simulink model "mpu6050_working"  (R2017a)
settings: Solver=FixedStepDiscrete  StartTime=0.0  StopTime=inf  RelTol=1e-3
PostLoadFcn:
  | ChipSelect = 1;  % choose I2C comms
  | AddressAlt = 0;  % use default address
  | 
  | if AddressAlt == 1
  | % b1101001 (pin AD0 is logic high).
  | SlvAddr = uint8(bin2dec('1101001'));  % ADDR ALT = 1
  | else
  | % b1101000 (pin AD0 is logic low)
  | SlvAddr = uint8(bin2dec('1101000'));  % ADDR ALT = 0
  | end
  | SlvAddr = uint8(hex2dec('68'));
  | 
  | 
  | % 0x3B 59 ACCEL_XOUT[15:8]
  | % 0x3C 60 ACCEL_XOUT[7:0]
  | % 0x3D 61 ACCEL_YOUT[15:8]
  | % 0x3E 62 ACCEL_YOUT[7:0]
  | % 0x3F 63 ACCEL_ZOUT[15:8]
  | % 0x40 64 ACCEL_ZOUT[7:0]
  | 
  | AccelXRegAddr = uint8(hex2dec('3B'));
  | AccelYRegAddr = uint8(hex2dec('3D'));
  | AccelZRegAddr = uint8(hex2dec('3F'));
  | 
  | % 0x43 67 GYRO_XOUT[15:8]
  | % 0x44 68 GYRO_XOUT[7:0]
  | % 0x45 69 GYRO_YOUT[15:8]
  | % 0x46 70 GYRO_YOUT[7:0]
  | % 0x47 71 GYRO_ZOUT[15:8]
  | % 0x48 72 GYRO_ZOUT[7:0]
  | 
  | GyroXRegAddr = uint8(hex2dec('43'));
  | GyroYRegAddr = uint8(hex2dec('45'));
  | GyroZRegAddr = uint8(hex2dec('47'));
  | 
  | deviceAddr = fi(SlvAddr,0,7,0);
  | 
  | powerRegAddr = uint8(hex2dec('6B'));
  | powerRegData = bin2dec('10000001');
undefined symbols (not defined in the file): fpgaClk, Ku, PWMFreq, Tu
libraries: simulink x1
settings Model: DataTypeOverride=Off  Creator=skuznick  LastModifiedBy=mini
settings DataIOCC: SaveOutput=off  SaveTime=off
settings OptimizationCC: BlockReduction=off  ConditionallyExecuteInputs=off  DefaultParameterBehavior=Inlined
settings DebuggingCC: AlgebraicLoopMsg=error  SingleTaskRateTransMsg=error
settings HardwareCC: ProdBitPerPointer=32  ProdBitPerSizeT=32  ProdBitPerPtrDiffT=32  ProdLargestAtomicFloat=None  ProdIntDivRoundTo=Undefined  ProdEndianess=Unspecified  ProdWordSize=32  ProdHWDeviceType=ASIC/FPGA->ASIC/FPGA  ProdEqTarget=off
settings GRTTargetCC: ExtMode=on

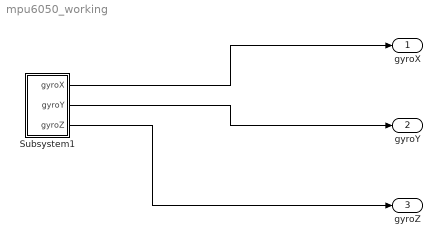
== system mpu6050_working ==
  Subsystem1 : Subsystem
  gyroX : Outport
  gyroY : Outport  Port=2
  gyroZ : Outport  Port=3
  wires:
  Subsystem1/1(gyroX) -> gyroX/1
  Subsystem1/2(gyroY) -> gyroY/1
  Subsystem1/3(gyroZ) -> gyroZ/1

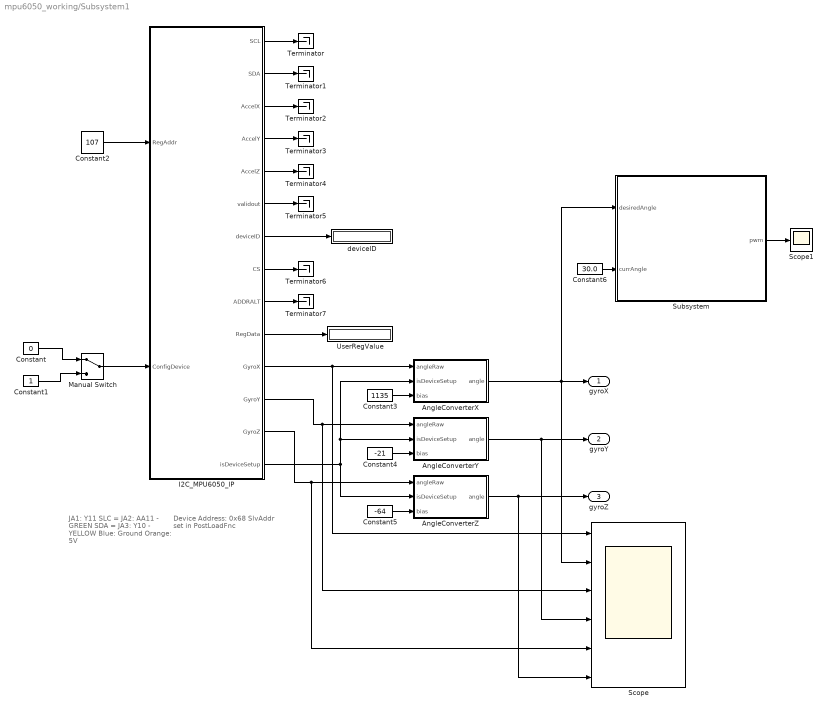
== system mpu6050_working/Subsystem1 ==
  note: JA1: Y11
      | SLC = JA2: AA11 - GREEN
      | SDA = JA3: Y10  - YELLOW
      | Blue: Ground
      | Orange: 5V
  note: Device Address: 0x68
      | SlvAddr set in PostLoadFnc
  AngleConverterX : Subsystem
  AngleConverterY : Subsystem
  AngleConverterZ : Subsystem
  Constant : Constant  Value=0  OutDataTypeStr=boolean  SampleTime=-1
  Constant1 : Constant  OutDataTypeStr=boolean  SampleTime=-1
  Constant2 : Constant  Value=107  OutDataTypeStr=uint8  SampleTime=-1
  Constant3 : Constant  Value=1135  OutDataTypeStr=int16
  Constant4 : Constant  Value=-21  OutDataTypeStr=int16
  Constant5 : Constant  Value=-64  OutDataTypeStr=int16
  Constant6 : Constant  Value=30.0  OutDataTypeStr=double
  I2C_MPU6050_IP : Subsystem  TreatAsAtomicUnit=on  SystemSampleTime=1/400e3
  Manual Switch : ManualSwitch
  Scope : Scope  NumInputPorts=6
  Scope1 : Scope
  Subsystem : Subsystem
  Terminator{,1..7} (8 alike) : Terminator
  UserRegValue : Display
  deviceID : Display
  gyroX : Outport
  gyroY : Outport  Port=2
  gyroZ : Outport  Port=3
  wires:
  I2C_MPU6050_IP/7(deviceID) -> deviceID/1
  Constant/1 -> Manual Switch/1
  Constant1/1 -> Manual Switch/2
  Constant2/1 -> I2C_MPU6050_IP/1(RegAddr)
  I2C_MPU6050_IP/10(RegData) -> UserRegValue/1
  Manual Switch/1 -> I2C_MPU6050_IP/2(ConfigDevice)
  I2C_MPU6050_IP/11(GyroX) -> Scope/1, AngleConverterX/1(angleRaw)
  I2C_MPU6050_IP/12(GyroY) -> Scope/3, AngleConverterY/1(angleRaw)
  Subsystem/1(pwm) -> Scope1/1
  I2C_MPU6050_IP/5(AccelZ) -> Terminator4/1
  AngleConverterZ/1(angle) -> gyroZ/1, Scope/6
  AngleConverterX/1(angle) -> gyroX/1, Subsystem/1(desiredAngle), Scope/2
  I2C_MPU6050_IP/4(AccelY) -> Terminator3/1
  I2C_MPU6050_IP/8(CS) -> Terminator6/1
  I2C_MPU6050_IP/9(ADDRALT) -> Terminator7/1
  Constant6/1 -> Subsystem/2(currAngle)
  I2C_MPU6050_IP/3(AccelX) -> Terminator2/1
  I2C_MPU6050_IP/6(validout) -> Terminator5/1
  I2C_MPU6050_IP/1(SCL) -> Terminator/1
  I2C_MPU6050_IP/2(SDA) -> Terminator1/1
  Constant4/1 -> AngleConverterY/3(bias)
  I2C_MPU6050_IP/14(isDeviceSetup) -> AngleConverterZ/2(isDeviceSetup), AngleConverterY/2(isDeviceSetup), AngleConverterX/2(isDeviceSetup)
  Constant5/1 -> AngleConverterZ/3(bias)
  Constant3/1 -> AngleConverterX/3(bias)
  I2C_MPU6050_IP/13(GyroZ) -> Scope/5, AngleConverterZ/1(angleRaw)
  AngleConverterY/1(angle) -> gyroY/1, Scope/4

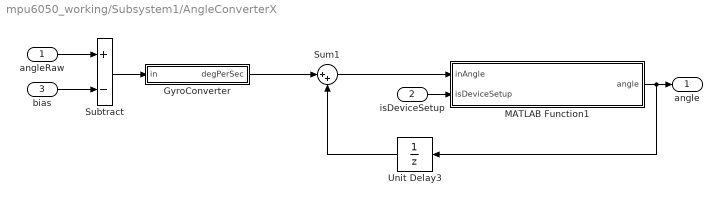
== system mpu6050_working/Subsystem1/AngleConverterX ==
  angleRaw : Inport  OutDataTypeStr=int16  Interpolate=off
  isDeviceSetup : Inport  Port=2  OutDataTypeStr=boolean  Interpolate=off
  bias : Inport  Port=3  OutDataTypeStr=int16  Interpolate=off
  GyroConverter : Subsystem
  MATLAB Function1 : MATLAB Function  TreatAsAtomicUnit=on
  Subtract : Sum  Inputs=+-  OutDataTypeStr=int16  SaturateOnIntegerOverflow=off  InputSameDT=off
  Sum1 : Sum  Inputs=|++  SaturateOnIntegerOverflow=off  InputSameDT=off  OutDataTypeStr=Inherit: Inherit via internal rule
  Unit Delay3 : UnitDelay  SampleTime=-1
  angle : Outport  OutDataTypeStr=double
  wires:
  MATLAB Function1/1(angle) -> Unit Delay3/1, angle/1
  isDeviceSetup/1 -> MATLAB Function1/2(isDeviceSetup)
  Sum1/1 -> MATLAB Function1/1(inAngle)
  Unit Delay3/1 -> Sum1/2
  GyroConverter/1(degPerSec) -> Sum1/1
  angleRaw/1 -> Subtract/1
  bias/1 -> Subtract/2
  Subtract/1 -> GyroConverter/1(in)

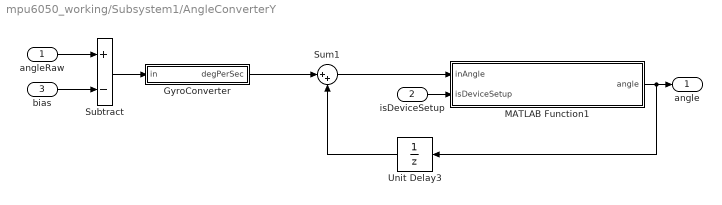
== system mpu6050_working/Subsystem1/AngleConverterY ==
  angleRaw : Inport  OutDataTypeStr=int16  Interpolate=off
  isDeviceSetup : Inport  Port=2  OutDataTypeStr=boolean  Interpolate=off
  bias : Inport  Port=3  OutDataTypeStr=int16  Interpolate=off
  GyroConverter : Subsystem
  MATLAB Function1 : MATLAB Function  TreatAsAtomicUnit=on
  Subtract : Sum  Inputs=+-  OutDataTypeStr=int16  SaturateOnIntegerOverflow=off  InputSameDT=off
  Sum1 : Sum  Inputs=|++  SaturateOnIntegerOverflow=off  InputSameDT=off  OutDataTypeStr=Inherit: Inherit via internal rule
  Unit Delay3 : UnitDelay  SampleTime=-1
  angle : Outport  OutDataTypeStr=double
  wires:
  MATLAB Function1/1(angle) -> Unit Delay3/1, angle/1
  isDeviceSetup/1 -> MATLAB Function1/2(isDeviceSetup)
  Sum1/1 -> MATLAB Function1/1(inAngle)
  Unit Delay3/1 -> Sum1/2
  GyroConverter/1(degPerSec) -> Sum1/1
  angleRaw/1 -> Subtract/1
  bias/1 -> Subtract/2
  Subtract/1 -> GyroConverter/1(in)

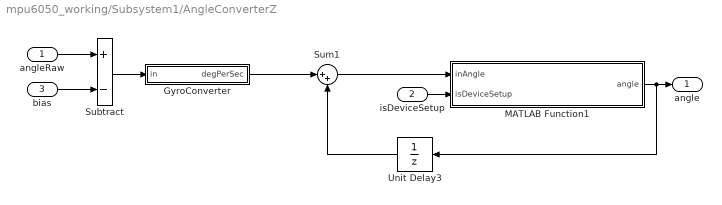
== system mpu6050_working/Subsystem1/AngleConverterZ ==
  angleRaw : Inport  OutDataTypeStr=int16  Interpolate=off
  isDeviceSetup : Inport  Port=2  OutDataTypeStr=boolean  Interpolate=off
  bias : Inport  Port=3  OutDataTypeStr=int16  Interpolate=off
  GyroConverter : Subsystem
  MATLAB Function1 : MATLAB Function  TreatAsAtomicUnit=on
  Subtract : Sum  Inputs=+-  OutDataTypeStr=int16  SaturateOnIntegerOverflow=off  InputSameDT=off
  Sum1 : Sum  Inputs=|++  SaturateOnIntegerOverflow=off  InputSameDT=off  OutDataTypeStr=Inherit: Inherit via internal rule
  Unit Delay3 : UnitDelay  SampleTime=-1
  angle : Outport  OutDataTypeStr=double
  wires:
  MATLAB Function1/1(angle) -> Unit Delay3/1, angle/1
  isDeviceSetup/1 -> MATLAB Function1/2(isDeviceSetup)
  Sum1/1 -> MATLAB Function1/1(inAngle)
  Unit Delay3/1 -> Sum1/2
  GyroConverter/1(degPerSec) -> Sum1/1
  angleRaw/1 -> Subtract/1
  bias/1 -> Subtract/2
  Subtract/1 -> GyroConverter/1(in)

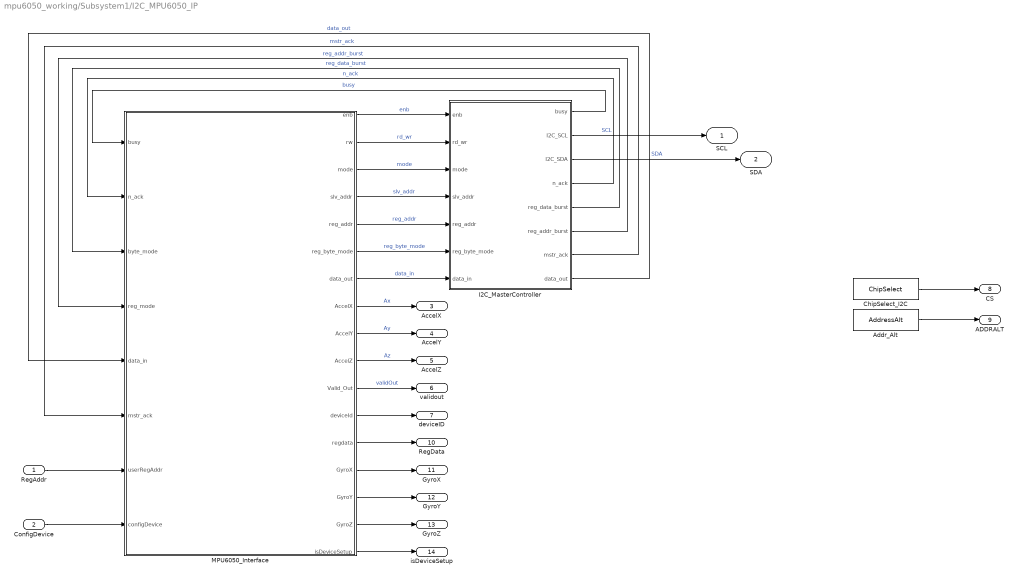
== system mpu6050_working/Subsystem1/I2C_MPU6050_IP ==
  RegAddr : Inport
  ConfigDevice : Inport  Port=2
  Addr_Alt : Constant  Value=AddressAlt  OutDataTypeStr=boolean  SampleTime=-1
  ChipSelect_I2C : Constant  Value=ChipSelect  OutDataTypeStr=boolean  SampleTime=-1
  I2C_MasterController : Subsystem
  MPU6050_Interface : Stateflow chart  TreatAsAtomicUnit=on
  SCL : Outport
  SDA : Outport  Port=2
  AccelX : Outport  Port=3
  AccelY : Outport  Port=4
  AccelZ : Outport  Port=5
  validout : Outport  Port=6
  deviceID : Outport  Port=7
  CS : Outport  Port=8
  ADDRALT : Outport  Port=9
  RegData : Outport  Port=10
  GyroX : Outport  Port=11
  GyroY : Outport  Port=12
  GyroZ : Outport  Port=13
  isDeviceSetup : Outport  Port=14
  wires:
  MPU6050_Interface/7(data_out) -> I2C_MasterController/7(data_in)  "data_in"
  I2C_MasterController/8(data_out) -> MPU6050_Interface/5(data_in)  "data_out"
  I2C_MasterController/7(mstr_ack) -> MPU6050_Interface/6(mstr_ack)  "mstr_ack"
  I2C_MasterController/4(n_ack) -> MPU6050_Interface/2(n_ack)  "n_ack"
  I2C_MasterController/5(reg_data_burst) -> MPU6050_Interface/3(byte_mode)  "reg_data_burst"
  I2C_MasterController/6(reg_addr_burst) -> MPU6050_Interface/4(reg_mode)  "reg_addr_burst"
  I2C_MasterController/1(busy) -> MPU6050_Interface/1(busy)  "busy"
  I2C_MasterController/3(I2C_SDA) -> SDA/1  "SDA"
  I2C_MasterController/2(I2C_SCL) -> SCL/1  "SCL"
  MPU6050_Interface/6(reg_byte_mode) -> I2C_MasterController/6(reg_byte_mode)  "reg_byte_mode"
  MPU6050_Interface/5(reg_addr) -> I2C_MasterController/5(reg_addr)  "reg_addr"
  MPU6050_Interface/4(slv_addr) -> I2C_MasterController/4(slv_addr)  "slv_addr"
  MPU6050_Interface/3(mode) -> I2C_MasterController/3(mode)  "mode"
  MPU6050_Interface/2(rw) -> I2C_MasterController/2(rd_wr)  "rd_wr"
  MPU6050_Interface/1(enb) -> I2C_MasterController/1(enb)  "enb"
  ChipSelect_I2C/1 -> CS/1
  Addr_Alt/1 -> ADDRALT/1
  MPU6050_Interface/9(AccelY) -> AccelY/1  "Ay"
  MPU6050_Interface/10(AccelZ) -> AccelZ/1  "Az"
  MPU6050_Interface/11(Valid_Out) -> validout/1  "validOut"
  MPU6050_Interface/8(AccelX) -> AccelX/1  "Ax"
  MPU6050_Interface/12(deviceId) -> deviceID/1
  MPU6050_Interface/13(regdata) -> RegData/1
  RegAddr/1 -> MPU6050_Interface/7(userRegAddr)
  MPU6050_Interface/14(GyroX) -> GyroX/1
  MPU6050_Interface/15(GyroY) -> GyroY/1
  MPU6050_Interface/16(GyroZ) -> GyroZ/1
  ConfigDevice/1 -> MPU6050_Interface/8(configDevice)
  MPU6050_Interface/17(isDeviceSetup) -> isDeviceSetup/1

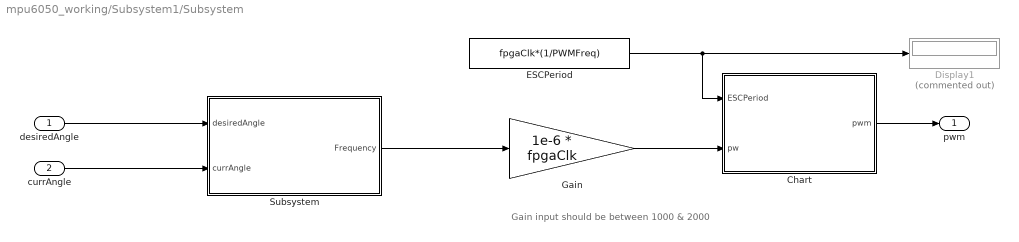
== system mpu6050_working/Subsystem1/Subsystem ==
  note: Gain input should be between 1000 & 2000
  desiredAngle : Inport
  currAngle : Inport  Port=2
  Chart : Stateflow chart  TreatAsAtomicUnit=on
  Display1 : Display  Commented=on
  ESCPeriod : Constant  Value=fpgaClk*(1/PWMFreq)  OutDataTypeStr=uint32
  Gain : Gain  Gain=1e-6 * fpgaClk  SaturateOnIntegerOverflow=off  ParamDataTypeStr=Inherit: Inherit via internal rule
  Subsystem : Subsystem
  pwm : Outport
  wires:
  Gain/1 -> Chart/2(pw)
  ESCPeriod/1 -> Chart/1(ESCPeriod), Display1/1
  Chart/1(pwm) -> pwm/1
  desiredAngle/1 -> Subsystem/1(desiredAngle)
  currAngle/1 -> Subsystem/2(currAngle)
  Subsystem/1(Frequency) -> Gain/1

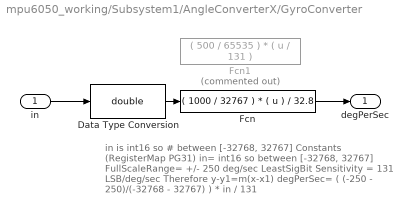
== system mpu6050_working/Subsystem1/AngleConverterX/GyroConverter ==
  note: in is int16 so # between [-32768, 32767]
      | Constants (RegisterMap PG31)
      | in= int16 so between [-32768, 32767]
      | FullScaleRange= +/- 250 deg/sec
      | LeastSigBit Sensitivity = 131 LSB/deg/sec
      | Therefore
      | y-y1=m(x-x1)
      | degPerSec= ( (-250 - 250)/(-32768 - 32767) ) * in / 131
  in : Inport  OutDataTypeStr=int16  Interpolate=off
  Data Type Conversion : DataTypeConversion  OutDataTypeStr=double  SaturateOnIntegerOverflow=off  RndMeth=Floor
  Fcn : Fcn  Expr=( 1000 / 32767 ) * ( u ) / 32.8
  Fcn1 : Fcn  Commented=on  Expr=( 500 / 65535 ) * ( u / 131 )
  degPerSec : Outport  OutDataTypeStr=double
  wires:
  Fcn/1 -> degPerSec/1
  in/1 -> Data Type Conversion/1
  Data Type Conversion/1 -> Fcn/1

== system mpu6050_working/Subsystem1/AngleConverterY/GyroConverter ==
  note: in is int16 so # between [-32768, 32767]
      | Constants (RegisterMap PG31)
      | in= int16 so between [-32768, 32767]
      | FullScaleRange= +/- 250 deg/sec
      | LeastSigBit Sensitivity = 131 LSB/deg/sec
      | Therefore
      | y-y1=m(x-x1)
      | degPerSec= ( (-250 - 250)/(-32768 - 32767) ) * in / 131
  in : Inport  OutDataTypeStr=int16  Interpolate=off
  Data Type Conversion : DataTypeConversion  OutDataTypeStr=double  SaturateOnIntegerOverflow=off  RndMeth=Floor
  Fcn : Fcn  Expr=( 1000 / 32767 ) * ( u )
  Fcn1 : Fcn  Commented=on  Expr=( 500 / 65535 ) * ( u / 131 )
  degPerSec : Outport  OutDataTypeStr=double
  wires:
  Fcn/1 -> degPerSec/1
  in/1 -> Data Type Conversion/1
  Data Type Conversion/1 -> Fcn/1

== system mpu6050_working/Subsystem1/AngleConverterZ/GyroConverter ==
  note: in is int16 so # between [-32768, 32767]
      | Constants (RegisterMap PG31)
      | in= int16 so between [-32768, 32767]
      | FullScaleRange= +/- 250 deg/sec
      | LeastSigBit Sensitivity = 131 LSB/deg/sec
      | Therefore
      | y-y1=m(x-x1)
      | degPerSec= ( (-250 - 250)/(-32768 - 32767) ) * in / 131
  in : Inport  OutDataTypeStr=int16  Interpolate=off
  Data Type Conversion : DataTypeConversion  OutDataTypeStr=double  SaturateOnIntegerOverflow=off  RndMeth=Floor
  Fcn : Fcn  Expr=( 1000 / 32767 ) * ( u )
  Fcn1 : Fcn  Commented=on  Expr=( 500 / 65535 ) * ( u / 131 )
  degPerSec : Outport  OutDataTypeStr=double
  wires:
  Fcn/1 -> degPerSec/1
  in/1 -> Data Type Conversion/1
  Data Type Conversion/1 -> Fcn/1

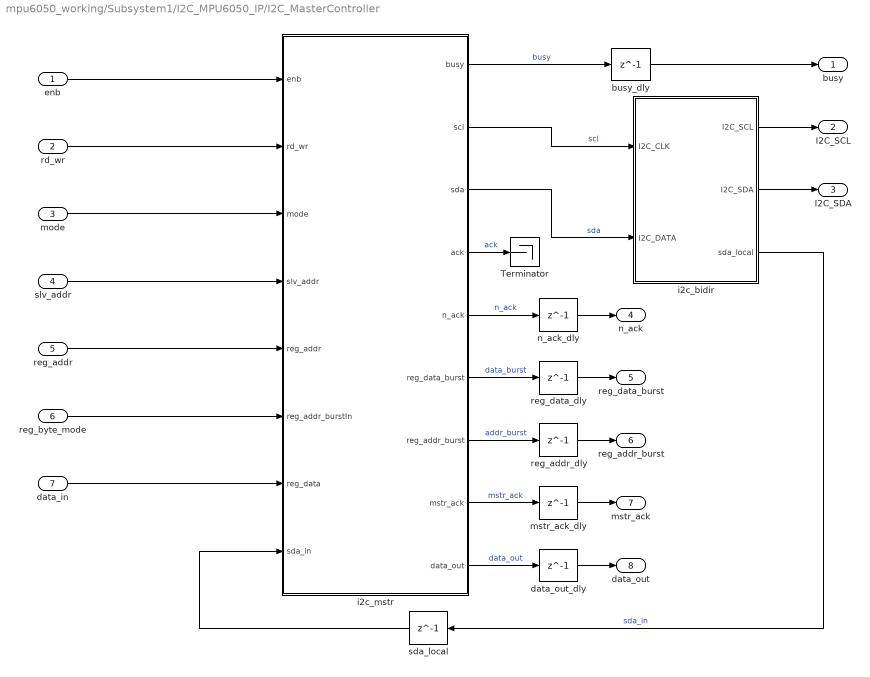
== system mpu6050_working/Subsystem1/I2C_MPU6050_IP/I2C_MasterController ==
  enb : Inport
  rd_wr : Inport  Port=2
  mode : Inport  Port=3
  slv_addr : Inport  Port=4
  reg_addr : Inport  Port=5
  reg_byte_mode : Inport  Port=6
  data_in : Inport  Port=7
  Terminator : Terminator
  busy_dly : Delay  DelayLength=1
  data_out_dly : Delay  DelayLength=1
  i2c_bidir : Subsystem  TreatAsAtomicUnit=on
  i2c_mstr : Stateflow chart  TreatAsAtomicUnit=on
  mstr_ack_dly : Delay  DelayLength=1
  n_ack_dly : Delay  DelayLength=1
  reg_addr_dly : Delay  DelayLength=1
  reg_data_dly : Delay  DelayLength=1
  sda_local : Delay  DelayLength=1
  busy : Outport
  I2C_SCL : Outport  Port=2
  I2C_SDA : Outport  Port=3
  n_ack : Outport  Port=4
  reg_data_burst : Outport  Port=5
  reg_addr_burst : Outport  Port=6
  mstr_ack : Outport  Port=7
  data_out : Outport  Port=8
  wires:
  data_out_dly/1 -> data_out/1
  mstr_ack_dly/1 -> mstr_ack/1
  i2c_mstr/9(data_out) -> data_out_dly/1  "data_out"
  i2c_mstr/8(mstr_ack) -> mstr_ack_dly/1  "mstr_ack"
  busy_dly/1 -> busy/1
  n_ack_dly/1 -> n_ack/1
  reg_data_dly/1 -> reg_data_burst/1
  reg_addr_dly/1 -> reg_addr_burst/1
  i2c_mstr/1(busy) -> busy_dly/1  "busy"
  rd_wr/1 -> i2c_mstr/2(rd_wr)
  mode/1 -> i2c_mstr/3(mode)
  data_in/1 -> i2c_mstr/7(reg_data)
  enb/1 -> i2c_mstr/1(enb)
  slv_addr/1 -> i2c_mstr/4(slv_addr)
  reg_byte_mode/1 -> i2c_mstr/6(reg_addr_burstIn)
  reg_addr/1 -> i2c_mstr/5(reg_addr)
  i2c_bidir/1(I2C_SCL) -> I2C_SCL/1
  i2c_bidir/2(I2C_SDA) -> I2C_SDA/1
  i2c_mstr/4(ack) -> Terminator/1  "ack"
  i2c_mstr/2(scl) -> i2c_bidir/1(I2C_CLK)  "scl"
  i2c_bidir/3(sda_local) -> sda_local/1  "sda_in"
  sda_local/1 -> i2c_mstr/8(sda_in)
  i2c_mstr/3(sda) -> i2c_bidir/2(I2C_DATA)  "sda"
  i2c_mstr/5(n_ack) -> n_ack_dly/1  "n_ack"
  i2c_mstr/6(reg_data_burst) -> reg_data_dly/1  "data_burst"
  i2c_mstr/7(reg_addr_burst) -> reg_addr_dly/1  "addr_burst"

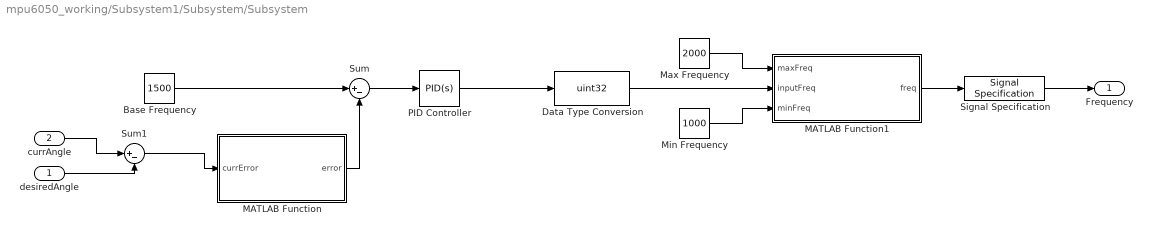
== system mpu6050_working/Subsystem1/Subsystem/Subsystem ==
  desiredAngle : Inport
  currAngle : Inport  Port=2
  Base Frequency : Constant  Value=1500
  Data Type Conversion : DataTypeConversion  OutDataTypeStr=uint32  SaturateOnIntegerOverflow=off  RndMeth=Floor
  MATLAB Function : MATLAB Function  TreatAsAtomicUnit=on
  MATLAB Function1 : MATLAB Function  TreatAsAtomicUnit=on
  Max Frequency : Constant  Value=2000  OutDataTypeStr=uint32
  Min Frequency : Constant  Value=1000  OutDataTypeStr=uint32
  PID Controller : simulink/Continuous/PID Controller  Controller=PID  TimeDomain=Continuous-time  SampleTime=-1  IntegratorMethod=Forward Euler  FilterMethod=Forward Euler  Form=Parallel  UseFilter=on  ControllerParametersSource=internal  P=0.6*Ku  I=1.2*Ku/Tu  D=0.6*Ku*Tu/8  N=100  InitialConditionSource=internal  InitialConditionForIntegrator=0  InitialConditionForFilter=0  ExternalReset=none  LimitOutput=off  UpperSaturationLimit=inf  LowerSaturationLimit=-inf  LinearizeAsGain=on  AntiWindupMode=none  Kb=1  TrackingMode=off  Kt=1  PParamMin=[]  PParamMax=[]  IParamMin=[]  IParamMax=[]  DParamMin=[]  DParamMax=[]  NParamMin=[]  NParamMax=[]  KbParamMin=[]  KbParamMax=[]  KtParamMin=[]  KtParamMax=[]  POutMin=[]  POutMax=[]  IOutMin=[]  IOutMax=[]  DOutMin=[]  DOutMax=[]  NOutMin=[]  NOutMax=[]  KbOutMin=[]  KbOutMax=[]  KtOutMin=[]  KtOutMax=[]  IntegratorOutMin=[]  IntegratorOutMax=[]  FilterOutMin=[]  FilterOutMax=[]  SumOutMin=[]  SumOutMax=[]  SumI1OutMin=[]  SumI1OutMax=[]  SumI2OutMin=[]  SumI2OutMax=[]  SumI3OutMin=[]  SumI3OutMax=[]  SumDOutMin=[]  SumDOutMax=[]  SaturationOutMin=[]  SaturationOutMax=[]  IntegratorContinuousStateAttributes=''  IntegratorStateMustResolveToSignalObject=off  IntegratorRTWStateStorageClass=Auto  FilterContinuousStateAttributes=''  FilterStateMustResolveToSignalObject=off  FilterRTWStateStorageClass=Auto  DifferentiatorICPrevScaledInput=0  DifferentiatorOutMin=[]  DifferentiatorOutMax=[]  InitialConditionSetting=State (most efficient)
  Signal Specification : SignalSpecification  OutDataTypeStr=uint32
  Sum : Sum  Inputs=|+-  SaturateOnIntegerOverflow=off  InputSameDT=off  OutDataTypeStr=Inherit: Inherit via internal rule
  Sum1 : Sum  Inputs=|+-  SaturateOnIntegerOverflow=off  InputSameDT=off  OutDataTypeStr=Inherit: Inherit via internal rule
  Frequency : Outport
  wires:
  Sum/1 -> PID Controller/1
  Base Frequency/1 -> Sum/1
  Min Frequency/1 -> MATLAB Function1/3(minFreq)
  Max Frequency/1 -> MATLAB Function1/1(maxFreq)
  desiredAngle/1 -> Sum1/2
  currAngle/1 -> Sum1/1
  MATLAB Function/1(error) -> Sum/2
  Sum1/1 -> MATLAB Function/1(currError)
  MATLAB Function1/1(freq) -> Signal Specification/1
  Signal Specification/1 -> Frequency/1
  PID Controller/1 -> Data Type Conversion/1
  Data Type Conversion/1 -> MATLAB Function1/2(inputFreq)

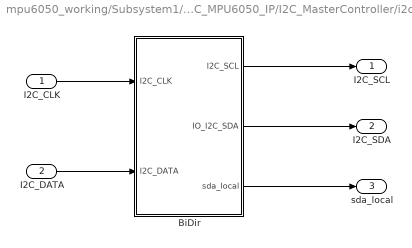
== system mpu6050_working/Subsystem1/I2C_MPU6050_IP/I2C_MasterController/i2c_bidir ==
  I2C_CLK : Inport
  I2C_DATA : Inport  Port=2
  BiDir : Subsystem  TreatAsAtomicUnit=on
  I2C_SCL : Outport
  I2C_SDA : Outport  Port=2
  sda_local : Outport  Port=3
  wires:
  BiDir/2(IO_I2C_SDA) -> I2C_SDA/1
  I2C_CLK/1 -> BiDir/1(I2C_CLK)
  I2C_DATA/1 -> BiDir/2(I2C_DATA)
  BiDir/1("I2C_SCL ") -> I2C_SCL/1
  BiDir/3(sda_local) -> sda_local/1

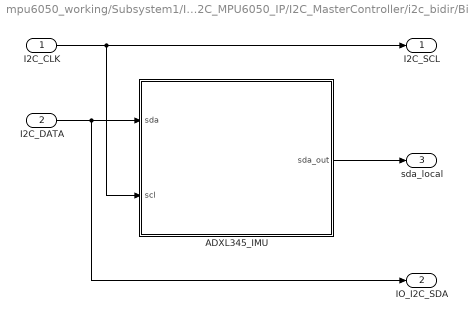
== system mpu6050_working/Subsystem1/I2C_MPU6050_IP/I2C_MasterController/i2c_bidir/BiDir ==
  I2C_CLK : Inport  OutDataTypeStr=boolean
  I2C_DATA : Inport  Port=2  OutDataTypeStr=boolean
  ADXL345_IMU : Stateflow chart  TreatAsAtomicUnit=on
  "I2C_SCL " : Outport  OutDataTypeStr=boolean
  IO_I2C_SDA : Outport  Port=2  OutDataTypeStr=boolean
  sda_local : Outport  Port=3  OutDataTypeStr=boolean
  wires:
  ADXL345_IMU/1(sda_out) -> sda_local/1
  I2C_CLK/1 -> "I2C_SCL "/1, ADXL345_IMU/2(scl)
  I2C_DATA/1 -> IO_I2C_SDA/1, ADXL345_IMU/1(sda)

== stateflow chart mpu6050_working/Subsystem1/I2C_MPU6050_IP/MPU6050_Interface ==
  settings: executeAtInitialization=1
  note: I2C Configuration for MPU6050
  note: 0x3B 59 ACCEL_XOUT[15:8]
      | 0x3C 60 ACCEL_XOUT[7:0]
      | 0x3D 61 ACCEL_YOUT[15:8]
      | 0x3E 62 ACCEL_YOUT[7:0]
      | 0x3F 63 ACCEL_ZOUT[15:8]
      | 0x40 64 ACCEL_ZOUT[7:0]
      |
      | 0x43 67 GYRO_XOUT[15:8]
      | 0x44 68 GYRO_XOUT[7:0]
      | 0x45 69 GYRO_YOUT[15:8]
      | 0x46 70 GYRO_YOUT[7:0]
      | 0x47 71 GYRO_ZOUT[15:8]
      | 0x48 72 GYRO_ZOUT[7:0]
      |
      | 0x6B 107 PWR_MGMT_1
      | 0x6C 108 PWR_MGMT_2
  state init
    %initstate
    Valid_Out = 0;
    isDeviceSetup = 1;
    slv_addr = SlvAddr;
  state idle
    %idlestate
    enb 	= 0;
    rw 		= 0;
    mode 	= 0;
    cnt      = 0;
    reg_byte_mode = 0;
  state Configuration [group]
    state setupReadWhoAmI
      entry:
      enb = 1;
      rw = 1;
      mode = 0;
      reg_addr = 117;
    state waitforNotBusy0
      enb=0;
    state readWhoAmI1
      %tmpData = uint8(data_in);
    state setupReadPwrMgmt1
      entry:
      enb = 1;
      rw = 1;
      mode = 0;
      reg_addr = 107;
    state waitforNotBusy1
      enb=0;
    state readPwrManagement1
      %tmpData = uint8(data_in);
    state setupFS_SEL
      enb = 1;
      rw = 0;
      mode = 0;
      reg_addr = 27; %0x1b
      data_out = 16; %fs range +/- 1000
    state waitforNotBusy3
      enb=0;
    state setupWritePwrMgmt1
      enb = 1;
      rw = 0;
      mode = 0;
      reg_addr = 107; %0x6B
      data_out = 0;
    state waitforNotBusy2
      enb=0;
    state cfgDone
      isDeviceSetup = 1;
    setupReadWhoAmI -> waitforNotBusy0 : [busy==1]
    waitforNotBusy0 -> (junction 2445) [order 1] : [n_ack==1]
    waitforNotBusy0 -> readWhoAmI1 [order 2] : [mstr_ack==1]
    readWhoAmI1 -> setupReadPwrMgmt1 : [busy==0]
    setupReadPwrMgmt1 -> Configuration.waitforNotBusy1 : [busy==1]
    Configuration.waitforNotBusy1 -> (junction 2445) [order 1] : [n_ack==1]
    Configuration.waitforNotBusy1 -> readPwrManagement1 [order 2] : [mstr_ack==1]
    readPwrManagement1 -> setupFS_SEL : [busy==0]
    setupFS_SEL -> waitforNotBusy3 : [busy==1]
    waitforNotBusy3 -> setupWritePwrMgmt1 [order 1] : [busy==0]
    waitforNotBusy3 -> (junction 2445) [order 2] : [n_ack==1]
    waitforNotBusy2 -> (junction 2445) [order 2] : [n_ack==1]
    setupWritePwrMgmt1 -> waitforNotBusy2 : [busy==1]
    waitforNotBusy2 -> cfgDone [order 1] : [busy==0]
  state ReadDeviceData [group]
    note: DEVID is an example of
        | doing a 1-byte READ
    note: 0x75 117 - WHO_AM_I[6:1]
    state getDEVID
      entry:
      enb = 1;
      rw = 1;
      mode = 0;
      reg_addr =   uint8(117);
    state waitforNotBusy1
      enb=0;
    state readDEVID
      deviceId = uint8(data_in);
    state debuggingState
      %tmp = 1
    state getRegData
      entry:
      enb = 1;
      rw = 1;
      mode = 0;
      reg_addr = userRegAddr;
    state waitforNotBusy5
      enb=0;
    state readUserRegData
      regdata = uint8(data_in);
    getDEVID -> ReadDeviceData.waitforNotBusy1 : [busy==1]
    ReadDeviceData.waitforNotBusy1 -> debuggingState [order 2] : [n_ack==1]
    ReadDeviceData.waitforNotBusy1 -> readDEVID [order 1] : [mstr_ack==1]
    readDEVID -> getRegData : [busy==0]
    debuggingState -> (junction 2281)
    getRegData -> waitforNotBusy5 : [busy==1]
    waitforNotBusy5 -> readUserRegData [order 1] : [mstr_ack==1]
    waitforNotBusy5 -> (junction 2281) [order 2] : [n_ack==1]
  state Valid
    en: enb = 0;
    cnt = 0;
    Valid_Out = 1;
    du: cnt = cnt + 1;
  state check_cfg
    en: enb = 0;
    cnt = 0;
    du: cnt = cnt + 1;
  state ReadGyroData [group]
    state setupReadGyroXoutH
      entry:
      enb = 1;
      rw = 1;
      mode = 0;
      reg_addr = 67; %0x43
    state waitforNotBusy06
      enb=0;
    state readGyroXoutH
      tempVal = uint8(data_in);
    state setupReadGyroXoutL
      entry:
      enb = 1;
      rw = 1;
      mode = 0;
      reg_addr = 68; %0x44
    state waitforNotBusy07
      enb=0;
    state readGyroXoutL
      GyroX = convert_int16(tempVal, data_in);;
    state setupReadGyroYoutH
      entry:
      enb = 1;
      rw = 1;
      mode = 0;
      reg_addr = 69; %0x45
    state waitforNotBusy04
      enb=0;
    state readGyroYoutH
      tempVal = uint8(data_in);
    state setupReadGyroYoutL
      entry:
      enb = 1;
      rw = 1;
      mode = 0;
      reg_addr = 70; %0x46
    state waitforNotBusy05
      enb=0;
    state readGyroYoutL
      GyroY = convert_int16(tempVal, data_in);
    state setupReadGyroZoutH
      entry:
      enb = 1;
      rw = 1;
      mode = 0;
      reg_addr = 71; %0x47
    state waitforNotBusy01
      enb=0;
    state readGyroZoutH
      tempVal = uint8(data_in);
    state setupReadGyroZoutL
      entry:
      enb = 1;
      rw = 1;
      mode = 0;
      reg_addr = 72; %0x48
    state waitforNotBusy03
      enb=0;
    state readGyroZoutL
      GyroZ = convert_int16(tempVal, data_in);
    setupReadGyroXoutH -> waitforNotBusy06 : [busy==1]
    waitforNotBusy06 -> (junction 2778) [order 2] : [n_ack==1]
    waitforNotBusy06 -> readGyroXoutH [order 1] : [mstr_ack==1]
    readGyroXoutH -> setupReadGyroXoutL : [busy==0]
    setupReadGyroXoutL -> waitforNotBusy07 : [busy==1]
    waitforNotBusy07 -> (junction 2778) [order 2] : [n_ack==1]
    waitforNotBusy07 -> readGyroXoutL [order 1] : [mstr_ack==1]
    readGyroXoutL -> setupReadGyroYoutH : [busy==0]
    waitforNotBusy04 -> (junction 2778) [order 2] : [n_ack==1]
    waitforNotBusy05 -> (junction 2778) [order 2] : [n_ack==1]
    waitforNotBusy01 -> (junction 2778) [order 2] : [n_ack==1]
    waitforNotBusy03 -> (junction 2778) [order 2] : [n_ack==1]
    setupReadGyroYoutH -> waitforNotBusy04 : [busy==1]
    waitforNotBusy04 -> readGyroYoutH [order 1] : [mstr_ack==1]
    readGyroYoutH -> setupReadGyroYoutL : [busy==0]
    setupReadGyroYoutL -> waitforNotBusy05 : [busy==1]
    waitforNotBusy05 -> ReadGyroData.readGyroYoutL [order 1] : [mstr_ack==1]
    ReadGyroData.readGyroYoutL -> setupReadGyroZoutH : [busy==0]
    setupReadGyroZoutH -> waitforNotBusy01 : [busy==1]
    waitforNotBusy01 -> readGyroZoutH [order 1] : [mstr_ack==1]
    readGyroZoutH -> setupReadGyroZoutL : [busy==0]
    setupReadGyroZoutL -> waitforNotBusy03 : [busy==1]
    waitforNotBusy03 -> readGyroZoutL [order 1] : [mstr_ack==1]
    readGyroZoutL -> (junction 2774) : [busy==0]
  state ReadAccelData [group]
    state setupReadAccelXoutH
      entry:
      enb = 1;
      rw = 1;
      mode = 0;
      reg_addr = 59; %0x3b
    state waitforNotBusya1
      enb=0;
    state readAccelXoutH
      tempVal = uint8(data_in);
    state setupReadAccelXoutL
      entry:
      enb = 1;
      rw = 1;
      mode = 0;
      reg_addr = 60; %0x3c
    state waitforNotBusya3
      enb=0;
    state readAccelXoutL
      AccelX = convert_int16(tempVal, data_in);
    state setupReadAccelYoutH
      entry:
      enb = 1;
      rw = 1;
      mode = 0;
      reg_addr = 61; %0x3d
    state waitforNotBusya4
      enb=0;
    state readAccelYoutH
      tempVal = uint8(data_in);
    state setupReadAccelYoutL
      entry:
      enb = 1;
      rw = 1;
      mode = 0;
      reg_addr = 62; %0x3e
    state waitforNotBusya5
      enb=0;
    state readGyroYoutL
      AccelY = convert_int16(tempVal, data_in);
    state setupReadAccelZoutH
      entry:
      enb = 1;
      rw = 1;
      mode = 0;
      reg_addr = 63; %0x3f
    state waitforNotBusya6
      enb=0;
    state readAccelZoutH
      tempVal = uint8(data_in);
    state setupReadAccelZoutL
      entry:
      enb = 1;
      rw = 1;
      mode = 0;
      reg_addr = 64; %0x40
    state waitforNotBusya7
      enb=0;
    state readAccelZoutL
      AccelZ = convert_int16(tempVal, data_in);
    setupReadAccelXoutH -> waitforNotBusya1 : [busy==1]
    waitforNotBusya1 -> (junction 2735) [order 2] : [n_ack==1]
    waitforNotBusya1 -> readAccelXoutH [order 1] : [mstr_ack==1]
    readAccelXoutH -> setupReadAccelXoutL : [busy==0]
    setupReadAccelXoutL -> waitforNotBusya3 : [busy==1]
    waitforNotBusya3 -> (junction 2735) [order 2] : [n_ack==1]
    waitforNotBusya3 -> readAccelXoutL [order 1] : [mstr_ack==1]
    readAccelXoutL -> setupReadAccelYoutH : [busy==0]
    waitforNotBusya4 -> (junction 2735) [order 2] : [n_ack==1]
    waitforNotBusya5 -> (junction 2735) [order 2] : [n_ack==1]
    waitforNotBusya6 -> (junction 2735) [order 2] : [n_ack==1]
    waitforNotBusya7 -> (junction 2735) [order 2] : [n_ack==1]
    setupReadAccelYoutH -> waitforNotBusya4 : [busy==1]
    waitforNotBusya4 -> readAccelYoutH [order 1] : [mstr_ack==1]
    readAccelYoutH -> setupReadAccelYoutL : [busy==0]
    setupReadAccelYoutL -> waitforNotBusya5 : [busy==1]
    waitforNotBusya5 -> ReadAccelData.readGyroYoutL [order 1] : [mstr_ack==1]
    ReadAccelData.readGyroYoutL -> setupReadAccelZoutH : [busy==0]
    setupReadAccelZoutH -> waitforNotBusya6 : [busy==1]
    waitforNotBusya6 -> readAccelZoutH [order 1] : [mstr_ack==1]
    readAccelZoutH -> setupReadAccelZoutL : [busy==0]
    setupReadAccelZoutL -> waitforNotBusya7 : [busy==1]
    waitforNotBusya7 -> readAccelZoutL [order 1] : [mstr_ack==1]
  (default) -> init
  init -> idle
  check_cfg -> idle : [cnt >=5]
  idle -> (junction 2460) : [busy==0]
  (junction 2460) -> setupReadWhoAmI [order 1] : [configDevice==1 | isDeviceSetup == 0]
  (junction 2460) -> getDEVID [order 2]
  (junction 2445) -> check_cfg
  readUserRegData -> setupReadAccelXoutH : [busy==0]
  (junction 2774) -> Valid
  (junction 2281) -> check_cfg
  Valid -> check_cfg : [cnt >= 5]
  (junction 2778) -> check_cfg
  (junction 2735) -> check_cfg
  cfgDone -> setupReadAccelXoutH
  readAccelZoutL -> setupReadGyroXoutH : [busy==0]
  data: msb function_input uint8; lsb function_input uint8; val function_output int16; enb output boolean size=1; rw output boolean size=1; mode output boolean; slv_addr output uint8; reg_addr output uint8; reg_byte_mode output boolean size=1; data_out output uint8; busy input; n_ack input; byte_mode input boolean size=1; reg_mode input boolean size=1; cnt local uint32; data_in input uint8 size=1; mstr_ack input; AccelX output int16; AccelY output int16; AccelZ output int16; SlvAddr parameter uint8; AccelXRegAddr parameter uint8; AccelYRegAddr parameter uint8; AccelZRegAddr parameter uint8; Valid_Out output boolean; tempVal local uint8; deviceId output uint8; powerRegData parameter uint8; regdata output uint8; userRegAddr input uint8; powerRegAddr parameter uint8; configDevice input boolean; GyroXRegAddr parameter uint8; GyroX output int16; GyroY output int16; GyroZ output int16; isDeviceSetup output boolean
  function val = convert_int16(msb, lsb):
    | function val = convert_int16(msb, lsb)
    | 
    | val = int16(bitor(bitshift(int16(msb),8), int16(lsb)));

== stateflow chart mpu6050_working/Subsystem1/I2C_MPU6050_IP/I2C_MasterController/i2c_mstr ==
  settings: executeAtInitialization=1
  state idle
    entry:
    scl(:) = 1;
    sda(:) = 1;
    busy(:)  = 0;
    reg_data_burst(:) = 0;
    temp_data = uint8(0);
  note: I2C Master Controller
  state stop_ext
    entry:
    scl (:) = 1;
    sda(:) = 1;
    ack(:) = 0;
  state ready
    entry:
    scl(:) = 1;
    sda(:) = 1;
    data_out(:) = 0;
  state stop
    entry:
    sda(:) = 0;
  state start_n
    entry:
    scl(:) = 1;
    sda(:) = 0;
    bit_cnt(:) = 7;
    busy(:) = 1;
    reg_byte_cnt =1;
    data_out(:) = 0;
  state mastr_ack_data_cnf1
    entry:
    scl(:) = 1;
    sda(:) = 1;
    mstr_ack (:) = 1;
  state mastr_ack_data_cnf
    entry:
    scl(:) = 1;
    sda(:) = 0;
    mstr_ack (:) = 1;
  state scl_ext_p
    entry:
    scl(:) = 1;
    sda(:) = 0;
    ack(:) = 0;
  state start_p
    entry:
    sda(:) = 0;
  state scl_ext_n
    entry:
    scl(:) = 0;
    sda(:) = 0;
    ack(:) = 0;
    mstr_ack(:) = 0;
  state mastr_ack_data
    entry:
    scl(:) = 0;
    if mode == 1
    sda(:) = 0; %ACK
    else
    sda(:) = 1; %NACK
    end
    mstr_ack(:) = 1;
    ack(:) = 0;
    data_out(:) = temp_data;
    temp_data(:) = 0;
  state cmd_slave_addr_n
    entry:
    scl(:) = 0;
    sda(:) = bitget(slv_addr(:),bit_cnt);
  state Increment_Byte_count1
    entry:
    scl(:) = 0;
    bit_cnt = 8;
    mstr_ack(:) =0;
    reg_data_burst(:) = 1;
    sda(:) = 1;
  state cmd_slave_addr_p
    entry:
    scl(:) = 1;
    bit_cnt = bit_cnt-1;
  state write_n
    entry:
    scl(:) = 0;
    sda(:) = 0;
  state ack_end1
    entry: scl(:)=1;
    sda(:)=1;
    ack(:)=1;
  state cmd_reg_read_data_p
    entry:
    scl(:) = 1;
    if sda_in == 1;
    temp_data = bitset(temp_data,bit_cnt);
    end
    bit_cnt = bit_cnt-1;
  state ack_end
    entry: scl(:)=1;
    sda(:)=1;
    ack(:)=1;
  state write_p
    entry:
    scl(:) = 1;
    sda(:) = 0;
  state ack_recv_wr3
    entry: scl(:)=1;
    sda(:)=1;
    ack(:)=1;
  state ack_data
    entry:
    scl(:) = 0;
    sda(:) = 1;
    ack(:) = 1;
  state ack_slv
    entry:
    scl(:) = 0;
    ack(:) = 1;
    sda(:) = 1;
  state cmd_reg_read_data_n
    entry:
    scl(:) = 0;
    %mstr_ack(:) = 0
    ack(:) = 1;
  state ack_recv_wr
    entry: scl(:)=1;
    sda(:)=1;
    ack(:)=1;
    bit_cnt = 8;
  state cmd_reg_data_p
    entry:
    scl(:) = 1;
    bit_cnt = bit_cnt-1;
  state ack_addr_m_cnf
    entry:
    scl(:) = 0;
    if rd_wr == 1
    sda(:) = 1;
    else
    sda(:) = 0;
    end
    bit_cnt = 8;
    ack(:) = 0;
  state ack_wr_p
    entry: scl(:)=0;
    ack(:)=0;
    sda(:)=0;
    bit_cnt = 8;
  state error_ack
    entry:
    scl(:) = 0;
    sda(:) = 1;
    n_ack(:) = 1;
  state cmd_reg_data_n
    entry:
    scl(:) = 0;
    ack(:) = 0;
    reg_data_burst(:) = 0;
    sda(:) = bitget(reg_data,bit_cnt);
  state delay
    entry:
    scl(:) = 0;
    sda(:) = 1;
  state cmd_reg_addr_n
    entry:
    scl(:) = 0;
    ack(:) = 0;
    sda(:) = bitget(reg_addr,bit_cnt);
    reg_addr_burst(:)=0;
  state repeat_strt_n
    entry:
    scl(:) = 1;
    sda(:) = 0;
    bit_cnt(:) = 7;
    busy(:) = 1;
    reg_byte_cnt =1;
  state ready_repeated
    entry:
    scl(:) = 1;
    sda(:) = 1;
  state cmd_reg_addr_p
    entry:
    scl(:)= 1;
    bit_cnt = bit_cnt-1;
  state repeat_strt_p
    entry:
    sda(:) = 0;
  state ready_repeated_dummy
    entry:
    scl(:) = 1;
    sda(:) = 1;
  state ack_addr_m
    entry:
    scl(:) = 0;
    ack (:) = 1;
    sda(:) = 1;
  state ack_recv_wr1
    entry: scl(:)=1;
    sda(:)=1;
    ack(:)=1;
  state ack_recv_wr2
    entry: scl(:)=1;
    sda(:)=1;
    ack(:)=1;
  state cmd_slave_addr_n1
    entry:
    scl(:) = 0;
    sda(:) = bitget(slv_addr(:),bit_cnt);
  state cmd_slave_addr_p1
    entry:
    scl(:) = 1;
    bit_cnt = bit_cnt-1;
  state ack_addrm1
    entry:
    scl(:) = 1;
    ack(:) = 0;
    bit_cnt = 8;
    reg_addr_burst(:)=1;
  state read_n
    entry:
    scl(:) = 0;
    sda(:) = 1;
  state ack_wr_p2
    entry: scl(:)=0;
    ack(:)=1;
    sda(:)=1;
  state read_p
    entry:
    scl(:) = 1;
    sda(:) = 1;
    bit_cnt = 8;
  state ack_slv1
    entry:
    scl(:) = 0;
    ack(:) = 1;
    sda(:) = 1;
  state ack_slv_cnf1
    entry:
    scl(:)= 1;
    ack(:) = 1;
    bit_cnt = 8;
  (default) -> idle
  stop_ext -> idle
  idle -> ready : [enb==1]
  stop -> stop_ext
  ready -> start_n
  scl_ext_p -> stop
  mastr_ack_data_cnf1 -> scl_ext_n
  start_n -> start_p
  mastr_ack_data_cnf -> Increment_Byte_count1
  mastr_ack_data -> mastr_ack_data_cnf [order 1] : [mode==1]
  mastr_ack_data -> mastr_ack_data_cnf1 [order 2]
  scl_ext_n -> scl_ext_p
  start_p -> cmd_slave_addr_n
  cmd_slave_addr_p -> cmd_slave_addr_n [order 1] : [bit_cnt > 0]
  error_ack -> scl_ext_n
  (junction 2294) -> scl_ext_n [order 2]
  cmd_slave_addr_n -> cmd_slave_addr_p
  cmd_slave_addr_p -> write_n [order 2]
  Increment_Byte_count1 -> cmd_reg_read_data_n
  ack_end -> (junction 2294) [order 1] : [sda_in == 0]
  (junction 2294) -> cmd_reg_data_n [order 1] : [mode == 1]{bit_cnt=8;reg_data_burst(:)=1;ack(:)=0;}
  cmd_reg_read_data_p -> mastr_ack_data [order 2]
  write_n -> write_p
  ack_data -> ack_end1
  ack_end1 -> ack_end
  cmd_reg_read_data_p -> cmd_reg_read_data_n [order 1] : [bit_cnt > 0]
  ack_slv -> ack_recv_wr3
  write_p -> ack_slv
  ack_end -> error_ack [order 2]
  cmd_reg_read_data_n -> cmd_reg_read_data_p
  ack_recv_wr3 -> ack_recv_wr
  cmd_reg_data_p -> ack_data [order 2]
  ack_wr_p2 -> cmd_reg_read_data_n
  ack_recv_wr -> error_ack [order 2]
  cmd_reg_data_p -> cmd_reg_data_n [order 1] : [bit_cnt > 0]
  ack_recv_wr -> ack_wr_p [order 1] : [sda_in == 0]
  cmd_reg_data_n -> cmd_reg_data_p
  ack_addr_m_cnf -> cmd_reg_data_n [order 1] : [rd_wr==0]
  ack_recv_wr2 -> ack_addr_m_cnf [order 1] : [sda_in == 0]
  ack_recv_wr2 -> error_ack [order 2]
  ack_slv_cnf1 -> error_ack [order 2]
  ack_wr_p -> cmd_reg_addr_n
  ack_addr_m_cnf -> delay [order 2] : [rd_wr==1]
  delay -> ready_repeated
  ack_addrm1 -> cmd_reg_addr_n
  cmd_reg_addr_p -> cmd_reg_addr_n [order 1] : [bit_cnt > 0]
  ready_repeated_dummy -> repeat_strt_n
  cmd_reg_addr_n -> cmd_reg_addr_p
  repeat_strt_n -> repeat_strt_p
  ready_repeated -> ready_repeated_dummy
  cmd_reg_addr_p -> ack_addr_m [order 2]
  repeat_strt_p -> cmd_slave_addr_n1
  ack_recv_wr1 -> ack_recv_wr2
  ack_addr_m -> ack_recv_wr1 [order 2]
  ack_addr_m -> ack_addrm1 [order 1] : [reg_addr_burstIn ==1]
  cmd_slave_addr_p1 -> cmd_slave_addr_n1 [order 1] : [bit_cnt > 0]
  cmd_slave_addr_n1 -> cmd_slave_addr_p1
  cmd_slave_addr_p1 -> read_n [order 2]
  read_n -> read_p
  ack_slv_cnf1 -> ack_wr_p2 [order 1] : [sda_in == 0]
  read_p -> ack_slv1
  ack_slv1 -> ack_slv_cnf1
  data: enb input boolean size=1; rd_wr input boolean size=1; mode input boolean size=1; busy output boolean size=1; bit_cnt local uint8; scl output boolean size=1; sda output boolean size=1; slv_addr input uint8; reg_addr input uint8; reg_addr_burstIn input boolean size=1; reg_data input uint8; sda_in input boolean size=1; ack output boolean size=1; n_ack output boolean size=1; reg_byte_cnt local uint8; reg_data_burst output boolean size=1; reg_addr_burst output boolean size=1; mstr_ack output boolean size=1; data_out output fixdt(0,8,0) size=1; temp_data local uint8

== matlab function mpu6050_working/Subsystem1/AngleConverterY/MATLAB Function1 ==
  data: inAngle input; angle output; isDeviceSetup input
function angle = fcn(inAngle, isDeviceSetup)
    if isDeviceSetup == true
        angle = inAngle;
    else
        angle = 0;
    end

== stateflow chart mpu6050_working/Subsystem1/I2C_MPU6050_IP/I2C_MasterController/i2c_bidir/BiDir/ADXL345_IMU ==
  state init
    entry:
    rd_cnt = 0;
    reg_idx = 0;
  state idle
    entry:
    sda_out = false;
    addr = fi(0,0,7,0);
    data = fi(0,0,8,0);
  state regdata = sendregdata(reg) [function]
    (default) -> (junction 86)
    (junction 86) -> (junction 89) [order 1] : [reg ==AccelXRegAddr]
    (junction 86) -> (junction 88) [order 2]
    (junction 89) -> (junction 90) : {regdata = hex2dec('D2');}
    (junction 90) -> (junction 99)
    (junction 99) -> (junction 112)
    (junction 88) -> (junction 97) [order 1] : [reg==AccelYRegAddr]
    (junction 97) -> (junction 111) : {regdata = hex2dec('E1');}
    (junction 88) -> (junction 91) [order 2]
    (junction 111) -> (junction 112)
    (junction 112) -> (junction 103)
    (junction 91) -> (junction 106) [order 1] : [reg==AccelZRegAddr]
    (junction 106) -> (junction 109) : {regdata=hex2dec('2E');}
    (junction 91) -> (junction 127) [order 2]
    (junction 109) -> (junction 103)
    (junction 103) -> (junction 143)
    (junction 127) -> (junction 126) [order 1] : [reg ==AccelXRegAddr+1]
    (junction 127) -> (junction 128) [order 2]
    (junction 126) -> (junction 131) : {regdata = hex2dec('04');}
    (junction 131) -> (junction 143)
    (junction 143) -> (junction 130)
    (junction 128) -> (junction 142) [order 1] : [reg==AccelYRegAddr+1]
    (junction 142) -> (junction 154) : {regdata = hex2dec('FF');}
    (junction 128) -> (junction 140) [order 2]
    (junction 154) -> (junction 130)
    (junction 130) -> (junction 149)
    (junction 140) -> (junction 141) [order 1] : [reg==AccelZRegAddr+1]
    (junction 141) -> (junction 153) : {regdata=hex2dec('16');}
    (junction 140) -> (junction 196) [order 2]
    (junction 153) -> (junction 149)
    (junction 149) -> (junction 197)
    (junction 196) -> (junction 194) [order 1] : [reg==powerRegAddr]
    (junction 194) -> (junction 192) : {regdata=hex2dec('FE');}
    (junction 196) -> (junction 152) [order 2] : {regdata=bin2dec('11100101');}
        | % Return the Device ID
    (junction 192) -> (junction 197)
    (junction 197) -> (junction 152)
  state start
    en:
    bit_idx(:) = 7;
  state startgetaddr
  state NACK
    entry: sda_out(:) = 1;
  state getaddr
    entry:
    if sda == 1
    addr = bitset(addr,bit_idx);
    end
    bit_idx = bit_idx - 1;
  note: RegX (0x32/0x33) = 1234 (0x04d2)
      | RegY (0x34/0x35) = 4321 (0x10e1)
      | RegZ (0x36/0x37) = 5678 (0x162e)
  state endgetaddr
    entry: rw = sda;
  state sendack
    entry:
    sda_out(:) = 0;
    bit_idx = 8;
  state senddatastart
    entry: data(:) = sendregdata(reg_idx+rd_cnt);
    bit_idx = 8;
  state waitForStop
  state getdatastart
  state sendbyte
    entry:
    sda_out(:) = bitget(data,bit_idx);
  state getdata
    entry:
    if sda == 1
    data = bitset(data,bit_idx);
    end
    bit_idx = bit_idx - 1;
  state sendbit
    entry:  bit_idx = bit_idx - 1;
  state waitforPos
  state endgetdata
    entry:
    reg_idx = uint8(data)
    sda_out(:) = 0;
  state lookRestart
    entry:
  state waitstop1
  state waitEndOfAck
  state getcfgregstart
  state sendAck
    entry: sda_out(:)=0;
    data
  state getcfgdata
    entry:
    if sda == 1
    data = bitset(data,bit_idx);
    end
    bit_idx = bit_idx - 1;
  (default) -> init
  init -> idle
  waitForStop -> idle : [scl==1 & sda==1]
  NACK -> idle
  idle -> start : [scl==1 & sda == 0]
  (junction 229) -> start [order 1] : [scl==1]
  start -> startgetaddr : [scl == 1]
  getaddr -> startgetaddr [order 1] : [bit_idx > 0]
  startgetaddr -> getaddr : [scl==1]
  endgetaddr -> NACK [order 1] : [addr ~= deviceAddr]
  getaddr -> endgetaddr [order 2] : [scl==1]
  endgetaddr -> sendack [order 2] : [scl==1]
  sendack -> senddatastart [order 1] : [scl==0 & rw==1]
  sendack -> getdatastart [order 2] : [scl==1 & rw==0] {rd_cnt=0;}
  waitstop1 -> senddatastart [order 2] : [scl==1&sda==0] {rd_cnt = rd_cnt + 1;}
  senddatastart -> sendbyte
  waitstop1 -> waitForStop [order 1] : [scl==1&sda==1]
  waitEndOfAck -> waitForStop : [scl==1&sda==0]
  getdata -> getdatastart [order 1] : [bit_idx > 0]
  getdatastart -> getdata : [scl == 1]
  sendbit -> sendbyte [order 1] : [bit_idx > 0]
  sendbyte -> sendbit : [scl==1]
  (junction 229) -> getcfgdata [order 2] : [scl==0] {bit_idx(:)=8;data(:)=0;}
  lookRestart -> (junction 229) : [sda==0]
  getdata -> endgetdata [order 2] : [scl==1]
  sendbit -> waitstop1 [order 2] : [scl==0]
  endgetdata -> waitforPos : [scl==1]
  waitforPos -> lookRestart [order 2] : [scl==1&sda==1]
  waitforPos -> getcfgdata [order 1] : [scl==1&sda==0] {bit_idx(:) = 8;
      |                 data(:) = 0;}
  sendAck -> waitEndOfAck : [scl==1]
  getcfgdata -> getcfgregstart [order 1] : [bit_idx > 0]
  getcfgregstart -> getcfgdata : [scl == 1]
  getcfgdata -> sendAck [order 2]
  data: reg function_input; regdata function_output; sda input boolean; scl input boolean; sda_out output boolean; addr local fixdt(0,7,0) size=1; bit_idx local uint8; deviceAddr parameter fixdt(0,7,0); data local fixdt(0,8,0) size=1; rw local boolean; reg_idx local uint8; rd_cnt local uint8; powerRegAddr parameter uint8; AccelXRegAddr parameter uint8; AccelYRegAddr parameter uint8; AccelZRegAddr parameter uint8

== matlab function mpu6050_working/Subsystem1/AngleConverterZ/MATLAB Function1 ==
  data: inAngle input; angle output; isDeviceSetup input
function angle = fcn(inAngle, isDeviceSetup)
    if isDeviceSetup == true
        angle = inAngle;
    else
        angle = 0;
    end

== stateflow chart mpu6050_working/Subsystem1/Subsystem/Chart ==
  settings: executeAtInitialization=1
  state on
    entry: cnt = uint32(0);
    pwm = true;
    during: cnt = cnt + 1;
  state off
    entry: pwm = false;
    during: cnt = cnt + 1;
  (default) -> on
  on -> off : [cnt > pw]
  off -> on : [cnt >= ESCPeriod]
  data: ESCPeriod input uint32; pw input uint32; pwm output boolean; cnt local uint32

== matlab function mpu6050_working/Subsystem1/Subsystem/Subsystem/MATLAB Function ==
  data: error output; currError input
function error = fcn(currError)
transError = -.01080*(currError)^3 + .678*(currError)^2 + 2.124*(currError) + 22.653;
if currError < 0
    error = transError * -1;
else
    error = transError;
end

== matlab function mpu6050_working/Subsystem1/Subsystem/Subsystem/MATLAB Function1 ==
  data: maxFreq input; inputFreq input; freq output uint32; minFreq input
function freq = fcn(maxFreq,inputFreq, minFreq)
    if( inputFreq > maxFreq ) 
        freq = maxFreq
    elseif ( inputFreq < minFreq ) 
        freq = minFreq
    else 
        freq = inputFreq
    end

== matlab function mpu6050_working/Subsystem1/AngleConverterX/MATLAB Function1 ==
  data: inAngle input; angle output; isDeviceSetup input
function angle = fcn(inAngle, isDeviceSetup)
    if isDeviceSetup == true
        angle = inAngle;
    else
        angle = 0;
    end
